simulink model "nspTimingGetNumPackets"  (R2012b)
settings: Solver=FixedStepDiscrete  StartTime=0.0  StopTime=10.0  FixedStep=0.001  RelTol=1e-3
libraries: xpclib x1
settings Model: BufferReuse=off  Creator=gilja  LastModifiedBy=Chethan
settings SolverCC: EnableConcurrentExecution=on  ConcurrentTasks=on
settings DataIOCC: SaveOutput=off  SignalLogging=off  SaveTime=off
settings OptimizationCC: InlineParams=on  InlineInvariantSignals=on  OptimizeBlockIOStorage=off  BufferReuse=off  ExpressionFolding=off  LocalBlockOutputs=off  SimCompilerOptimization=On
settings HardwareCC: ProdIntDivRoundTo=Zero  ProdEndianess=LittleEndian  ProdHWDeviceType=Generic->32-bit x86 compatible
settings ModelReferenceCC: ModelReferenceNumInstancesAllowed=Single  ModelReferenceMinAlgLoopOccurrences=on
settings RTWCC: SystemTargetFile=xpctarget.tlc  TemplateMakefile=xpc_default_tmf  Description=xPC Target  ProcessScript=xpctarget_make_rtw_hook  RTWCompilerOptimization=On
settings CodeAppCC: MaxIdLength=62
settings xpcTargetCC: TargetFcnLib=ansi_tfl_table_tmw.mat  CodeReplacementLibrary=XPC_BLAS  ParMdlRefBuildCompliant=on  ConcurrentExecutionCompliant=on  CombineSignalStateStructs=off  GRTInterface=on  xPCTaskExecutionProfile=on  xPCRL32EventNumber=5000  xPCisDownloadable=off  xPCLoadParamSetFile=off  xPCConcurrentTasks=off  xPCEnableSFAnimation=off

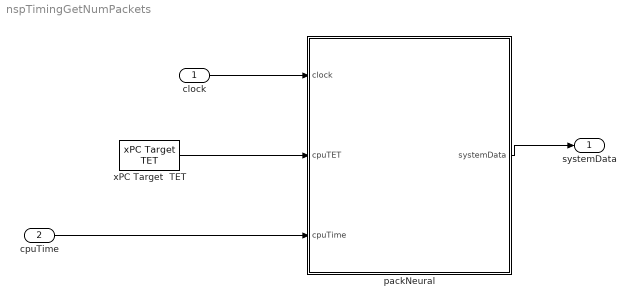
== system nspTimingGetNumPackets ==
  clock : Inport  OutDataTypeStr=uint32
  cpuTime : Inport  Port=2  OutDataTypeStr=uint32
  packNeural : MATLAB Function  TreatAsAtomicUnit=on
  "xPC Target  TET " : xpclib/Misc./xPC Target  TET   ts=0.001
  systemData : Outport  OutDataTypeStr=Bus: fileLoggerFormatAndData  BusOutputAsStruct=on
  wires:
  clock/1 -> packNeural/1(clock)
  packNeural/1(systemData) -> systemData/1
  cpuTime/1 -> packNeural/3(cpuTime)
  "xPC Target  TET "/1 -> packNeural/2(cpuTET)

== matlab function nspTimingGetNumPackets/packNeural ==
  data: systemData output Bus: fileLoggerFormatAndData size=1; clock input; cpuTET input; cpuTime input
function systemData = packNeural(clock, cpuTET, cpuTime)
%#codegen

VERSION_ID = single(1.1);

outputstring = 'system';

%% PACK DATA FOR UDP OUTPUT
systemData = packFileLoggerFormatAndData(outputstring, ...
    'systemDataPackage', VERSION_ID, ...
    'clock', clock, ...
    'cpuTET', cpuTET, ...
    'cpuTimes', cpuTime ...
    );

systemData.data.send = true;
